simulink model "Main"  (R2016b)
settings: Solver=ode45  StartTime=0.0  StopTime=t_end  FixedStep=st  MaxStep=st  RelTol=1e-3  EnableMultiTasking=on
values from neighbouring files (symbols this model uses):
  A = eye(16,16)    [full_input_list.m]
  counter = 0    [full_input_list.m]
  I_1 = [m*(zl^2+xyl^2)/12 0 0 ;          0 m*(zl^2+xyl^2)/12 0 ;          0 0 m*(2*xyl^2)/12 ] + 1e-6*(rand(3)-0.5)    [initACS.m]
  I_1_inv = inv(I_1)    [initACS.m]
  I_2 = [m*(zl^2+xyl^2)/12 0 0 ;          0 m*(zl^2+xyl^2)/12 0 ;          0 0 m*(2*xyl^2)/12 ] + 1e-6*(rand(3)-0.5)    [initACS.m]
  I_2_inv = inv(I_2)    [initACS.m]
  I_3 = [m*(zl^2+xyl^2)/12 0 0 ;          0 m*(zl^2+xyl^2)/12 0 ;          0 0 m*(2*xyl^2)/12 ] + 1e-6*(rand(3)-0.5)    [initACS.m]
  I_3_inv = inv(I_3)    [initACS.m]
  kd = 0.5    [full_input_list.m]    (also in initACS.m = 0.01)
  kp = 1    [full_input_list.m]    (also in initACS.m = 0.01)
  OpModes = [0 0 0]    [full_input_list.m]
  OpTimes = [0 1 2]    [full_input_list.m]
  SeperationTime = 30000    [full_input_list.m]
  state1_i = [ 0 0 0 , 0 0 0 , q4_0', w0_N]'    [full_input_list.m]
  state2_i = [ 0 0 (teth_length+side1Dim(1)/2+centerDim(3)/2+10*eps) , 0 -.1 0 ,      q4_0_Cube2' , w0_N ]'    [full_input_list.m]
  state3_i = [ 0 0 -(teth_length+side1Dim(1)/2+centerDim(3)/2+10*eps), 0 .1 0 ,      q4_0_Cube3' , w0_N ]'    [full_input_list.m]
  teth_k = teth_area*teth_modulus/teth_length    (= 33772.1210261)    [full_input_list.m]    (also in initACS.m = 10)
  teth_lo = 30    [full_input_list.m]    (also in initACS.m)
undefined symbols (not defined in the file or in its folder): DiscIntNeverNeededParam, Inertia, km, n, SolarDeployTime, solarpanel1_i, solarpanel2_i
libraries: SimMainLibrary x11, aerolibutil x10, simulink x1, vrlib x1, dspmathops x1
(part 2 of 2)

== matlab function Main/Flight Computers/MainCubeController/Navigation/Torque Coil Management/I_PWMOutput Function ==
  data: I_des input; pwm output; t input; dir output
function [pwm, dir] = fcn(I_des,t)
% max voltage is 3.3V. limit in current is depedent on coil location:
% 0.8A for Iz, and 0.2A for Ix and Iy. An internal power computation has
% to be performed to ensure that the power consumption of the coils is no
% more than 3W.
    I_maxZ = 0.2;
    I_maxYX = 0.8;
    I_max = [I_maxYX; I_maxYX; I_maxZ]; % limits power output of the coils
                                        % for a total of 3W of power at
                                        % 3.3V
    if max(I_max) == I_maxYX
        I_max = I_max/2 + [0;0;I_maxZ/2];
    end
    I_magn = abs(I_des);    % outputs the unsigned magnitude of each I component
    dir = sign(I_des);      % outputs direction of current flow needed
    
    del_t = min(I_magn,  I_max)/I_max;
    pwm = del_t;
end
